simulink model "Control_Block_Ke"  (R2020a)
settings: Solver=VariableStepAuto  StartTime=0.0  StopTime=10.0  RelTol=1e-3
libraries: fuzblock x5
settings Model: Creator=chris  LastModifiedBy=chris

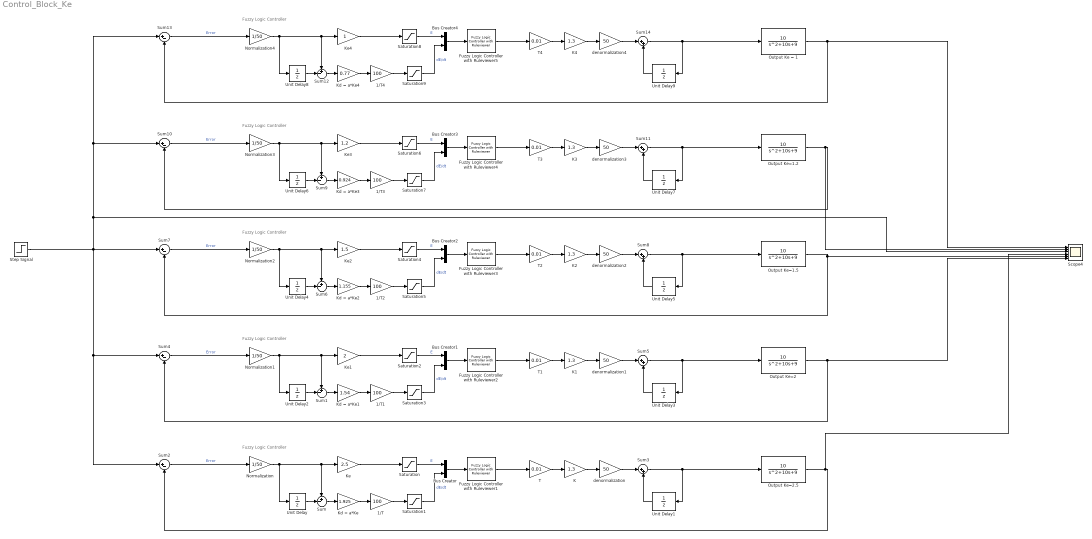
== system Control_Block_Ke ==
  note: Fuzzy Logic Controller
  note: Fuzzy Logic Controller
  note: Fuzzy Logic Controller
  note: Fuzzy Logic Controller
  note: Fuzzy Logic Controller
  1/T{,1..4} (5 alike) : Gain  Gain=100
  Bus Creator{,1..4} (5 alike) : BusCreator  Inputs=2
  Fuzzy Logic Controller with Ruleviewer{1..5} (5 alike) : fuzblock/Fuzzy Logic  Controller  with Ruleviewer  fismatrix=FLC  Ts=0.01
  K{,1..4} (5 alike) : Gain  Gain=1.3
  Kd = a*Ke : Gain  Gain=1.925
  Kd = a*Ke1 : Gain  Gain=1.54
  Kd = a*Ke2 : Gain  Gain=1.155
  Kd = a*Ke3 : Gain  Gain=0.924
  Kd = a*Ke4 : Gain  Gain=0.77
  Ke : Gain  Gain=2.5
  Ke1 : Gain  Gain=2
  Ke2 : Gain  Gain=1.5
  Ke3 : Gain  Gain=1.2
  Ke4 : Gain
  Normalization{,1..4} (5 alike) : Gain  Gain=1/50
  Output Ke = 1 : TransferFcn  Numerator=[10]  Denominator=[1 10 9]
  Output Ke=1.2 : TransferFcn  Numerator=[10]  Denominator=[1 10 9]
  Output Ke=1.5 : TransferFcn  Numerator=[10]  Denominator=[1 10 9]
  Output Ke=2 : TransferFcn  Numerator=[10]  Denominator=[1 10 9]
  Output Ke=2.5 : TransferFcn  Numerator=[10]  Denominator=[1 10 9]
  Saturation{,1..9} (10 alike) : Saturate  UpperLimit=1  LowerLimit=-1
  Scope4 : Scope  NumInputPorts=6
  Step Signal : Step  Time=0  After=50  SampleTime=0.01
  Sum{,1,6,9,12} (5 alike) : Sum  Inputs=+-|
  Sum{2,4,7,10,13} (5 alike) : Sum  Inputs=|+-
  Sum{3,5,8,11,14} (5 alike) : Sum  Inputs=|++
  T{,1..4} (5 alike) : Gain  Gain=0.01
  Unit Delay{,1..9} (10 alike) : UnitDelay  SampleTime=-1  HasFrameUpgradeWarning=on
  denormalization{,1..4} (5 alike) : Gain  Gain=50
  wires:
  Bus Creator/1 -> Fuzzy Logic Controller with Ruleviewer1/1
  Fuzzy Logic Controller with Ruleviewer1/1 -> T/1
  Normalization/1 -> Ke/1, Sum/1, Unit Delay/1
  Ke/1 -> Saturation/1
  T/1 -> K/1
  Saturation1/1 -> Bus Creator/2  "dE/dt"
  Kd = a*Ke/1 -> 1/T/1
  denormalization/1 -> Sum3/1
  Unit Delay/1 -> Sum/2
  Sum/1 -> Kd = a*Ke/1
  Saturation/1 -> Bus Creator/1  "E"
  Unit Delay1/1 -> Sum3/2
  K/1 -> denormalization/1
  1/T/1 -> Saturation1/1
  Output Ke=2.5/1 -> Scope4/4, Sum2/2
  Sum3/1 -> Unit Delay1/1, Output Ke=2.5/1
  Sum2/1 -> Normalization/1  "Error"
  Sum5/1 -> Unit Delay3/1, Output Ke=2/1
  Ke1/1 -> Saturation2/1
  K1/1 -> denormalization1/1
  1/T1/1 -> Saturation3/1
  Saturation3/1 -> Bus Creator1/2  "dE/dt"
  Unit Delay3/1 -> Sum5/2
  Output Ke=2/1 -> Scope4/6, Sum4/2
  Normalization1/1 -> Ke1/1, Sum1/1, Unit Delay2/1
  Sum1/1 -> Kd = a*Ke1/1
  Saturation2/1 -> Bus Creator1/1  "E"
  Unit Delay2/1 -> Sum1/2
  Bus Creator1/1 -> Fuzzy Logic Controller with Ruleviewer2/1
  Kd = a*Ke1/1 -> 1/T1/1
  Sum4/1 -> Normalization1/1  "Error"
  denormalization1/1 -> Sum5/1
  Fuzzy Logic Controller with Ruleviewer2/1 -> T1/1
  T1/1 -> K1/1
  Sum8/1 -> Unit Delay5/1, Output Ke=1.5/1
  Ke2/1 -> Saturation4/1
  K2/1 -> denormalization2/1
  1/T2/1 -> Saturation5/1
  Saturation5/1 -> Bus Creator2/2  "dE/dt"
  Unit Delay5/1 -> Sum8/2
  Output Ke=1.5/1 -> Sum7/2, Scope4/5
  Normalization2/1 -> Ke2/1, Sum6/1, Unit Delay4/1
  Sum6/1 -> Kd = a*Ke2/1
  Saturation4/1 -> Bus Creator2/1  "E"
  Unit Delay4/1 -> Sum6/2
  Bus Creator2/1 -> Fuzzy Logic Controller with Ruleviewer3/1
  Kd = a*Ke2/1 -> 1/T2/1
  Sum7/1 -> Normalization2/1  "Error"
  denormalization2/1 -> Sum8/1
  Fuzzy Logic Controller with Ruleviewer3/1 -> T2/1
  T2/1 -> K2/1
  Sum11/1 -> Unit Delay7/1, Output Ke=1.2/1
  Ke3/1 -> Saturation6/1
  K3/1 -> denormalization3/1
  1/T3/1 -> Saturation7/1
  Saturation7/1 -> Bus Creator3/2  "dE/dt"
  Unit Delay7/1 -> Sum11/2
  Output Ke=1.2/1 -> Scope4/2, Sum10/2
  Normalization3/1 -> Ke3/1, Sum9/1, Unit Delay6/1
  Sum9/1 -> Kd = a*Ke3/1
  Saturation6/1 -> Bus Creator3/1  "E"
  Unit Delay6/1 -> Sum9/2
  Bus Creator3/1 -> Fuzzy Logic Controller with Ruleviewer4/1
  Kd = a*Ke3/1 -> 1/T3/1
  Sum10/1 -> Normalization3/1  "Error"
  denormalization3/1 -> Sum11/1
  Fuzzy Logic Controller with Ruleviewer4/1 -> T3/1
  T3/1 -> K3/1
  Sum14/1 -> Unit Delay9/1, Output Ke = 1/1
  Ke4/1 -> Saturation8/1
  K4/1 -> denormalization4/1
  1/T4/1 -> Saturation9/1
  Saturation9/1 -> Bus Creator4/2  "dE/dt"
  Unit Delay9/1 -> Sum14/2
  Output Ke = 1/1 -> Sum13/2, Scope4/1
  Normalization4/1 -> Ke4/1, Sum12/1, Unit Delay8/1
  Sum12/1 -> Kd = a*Ke4/1
  Saturation8/1 -> Bus Creator4/1  "E"
  Unit Delay8/1 -> Sum12/2
  Bus Creator4/1 -> Fuzzy Logic Controller with Ruleviewer5/1
  Kd = a*Ke4/1 -> 1/T4/1
  Sum13/1 -> Normalization4/1  "Error"
  denormalization4/1 -> Sum14/1
  Fuzzy Logic Controller with Ruleviewer5/1 -> T4/1
  T4/1 -> K4/1
  Step Signal/1 -> Sum2/1, Sum4/1, Scope4/3, Sum10/1, Sum13/1, Sum7/1
